simulink model "chute_libre"  (R2016a)
settings: Solver=VariableStepAuto  StartTime=0.0  StopTime=10.0  RelTol=1e-3
libraries: simulink x1
settings Model: Creator=tmeunier  LastModifiedBy=tmeunier

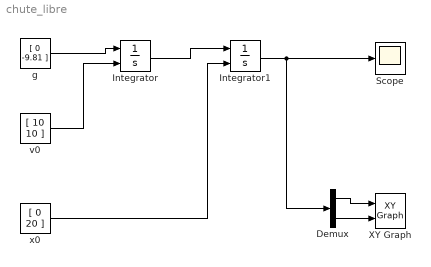
== system chute_libre ==
  Demux : Demux  Outputs=2
  Integrator : Integrator  InitialConditionSource=external
  Integrator1 : Integrator  InitialConditionSource=external
  Scope : Scope
  XY Graph : simulink/Sinks/XY Graph  xmin=0  xmax=100  ymin=-400  ymax=50  st=-1
  g : Constant  Value=[ 0 -9.81 ]
  v0 : Constant  Value=[ 10 10 ]
  x0 : Constant  Value=[ 0 20 ]
  wires:
  g/1 -> Integrator/1
  v0/1 -> Integrator/2
  Integrator/1 -> Integrator1/1
  x0/1 -> Integrator1/2
  Demux/1 -> XY Graph/1
  Demux/2 -> XY Graph/2
  Integrator1/1 -> Demux/1, Scope/1
